simulink model "link"  (R2025b)
settings: Solver=FixedStepAuto  StartTime=0.0  StopTime=10.0  RelTol=1e-3
undefined symbols (not defined in the file): link_params, Ts_inner
settings Model: DataDictionary=project.sldd  Creator=Nick  LastModifiedBy=Nick

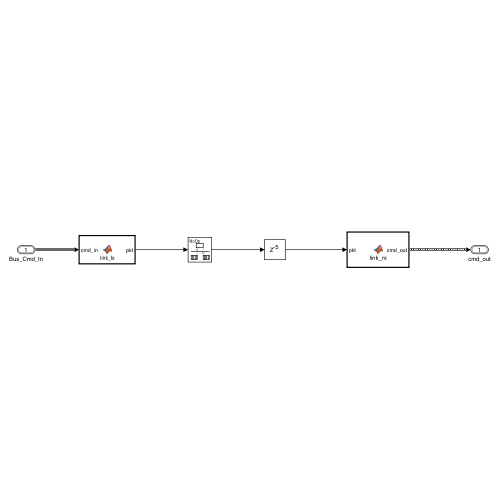
[thumbnail: Simulink's stored preview of the top-level diagram]
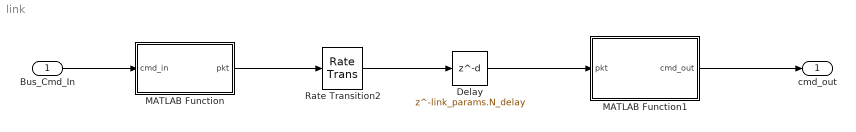
== system link ==
  Bus_Cmd_In : Inport  OutDataTypeStr=Bus: Bus_Cmd
  Delay : Delay  DelayLength=link_params.N_delay  InitialCondition=link_params.pkt_init_delay  SampleTime=Ts_inner
  MATLAB Function : MATLAB Function  TreatAsAtomicUnit=on
  MATLAB Function1 : MATLAB Function  TreatAsAtomicUnit=on
  Rate Transition2 : RateTransition  OutPortSampleTime=Ts_sim
  cmd_out : Outport  OutDataTypeStr=Bus: Bus_Cmd
  wires:
  Bus_Cmd_In/1 -> MATLAB Function/1(cmd_in)
  MATLAB Function/1(pkt) -> Rate Transition2/1
  Rate Transition2/1 -> Delay/1
  Delay/1 -> MATLAB Function1/1(pkt)
  MATLAB Function1/1(cmd_out) -> cmd_out/1

== matlab function link/MATLAB Function1 ==
  data: pkt input int16 size=[19 1]; link_params parameter; cmd_out output Bus: Bus_Cmd
function cmd_out = link_rx(pkt, link_params)
%#codegen
% RX-Seite Funkkanal (Drohne) @ Ts_inner.
%   int16-Paket (19x1) -> dequantisieren -> Bus_Cmd
%   Quaternionen werden re-normiert (Quant-Rauschen entfernen).
p    = reshape(double(pkt), 19, 1);
fs   = reshape(double(link_params.fs), 19, 1);
qmax = double(link_params.qmax);
lsb  = fs / qmax;
v    = reshape(p .* lsb, 19, 1);
F    = v(1);
qd   = reshape(v(2:5),   4, 1);
qr   = reshape(v(6:9),   4, 1);
Om   = reshape(v(10:12), 3, 1);
tr   = reshape(v(13:15), 3, 1);
qe   = reshape(v(16:19), 4, 1);
n_qd = sqrt(qd.'*qd); if n_qd < 1e-12, n_qd = 1; end
n_qr = sqrt(qr.'*qr); if n_qr < 1e-12, n_qr = 1; end
n_qe = sqrt(qe.'*qe); if n_qe < 1e-12, n_qe = 1; end
cmd_out.F_des     = F;
cmd_out.q_des     = qd / n_qd;
cmd_out.q_ref     = qr / n_qr;
cmd_out.Omega_ref = Om;
cmd_out.tau_ref   = tr;
cmd_out.q_ext     = qe / n_qe;
end

== matlab function link/MATLAB Function ==
  data: cmd_in input Bus: Bus_Cmd; pkt output int16 size=[19 1]; link_params parameter
function pkt = link_tx(cmd_in, link_params)
%#codegen
% TX-Seite Funkkanal (GCS->Drohne) @ Ts_gcs.
%   (1) Bus_Cmd -> 19x1 double in fester Reihenfolge packen
%   (2) int16-Quantisierung mit Saturierung
%   (3) Bernoulli-Paketverlust (xorshift32); bei Verlust letztes Paket halten (ZOH).
persistent last_pkt rs init_done
if isempty(init_done)
    last_pkt  = reshape(int16(link_params.pkt_init), 19, 1);
    rs        = uint32(link_params.seed);
    init_done = true;
end
F   = double(cmd_in.F_des);
qd  = reshape(double(cmd_in.q_des),     4, 1);
qr  = reshape(double(cmd_in.q_ref),     4, 1);
Om  = reshape(double(cmd_in.Omega_ref), 3, 1);
tr  = reshape(double(cmd_in.tau_ref),   3, 1);
qe  = reshape(double(cmd_in.q_ext),     4, 1);
v   = reshape([F; qd; qr; Om; tr; qe], 19, 1);
fs   = reshape(double(link_params.fs), 19, 1);
qmax = double(link_params.qmax);
qmin = double(link_params.qmin);
lsb  = fs / qmax;
qi      = min(max(round(v ./ lsb), qmin), qmax);
pkt_now = reshape(int16(qi), 19, 1);
[u, rs] = xorshift01(rs);
if u >= link_params.pdrop
    last_pkt = pkt_now;
end
pkt = reshape(last_pkt, 19, 1);
end
function [u, s] = xorshift01(s)
% xorshift32 -> u in [0,1). Seed != 0 erforderlich.
s = bitxor(s, bitshift(s,  13));
s = bitxor(s, bitshift(s, -17));
s = bitxor(s, bitshift(s,   5));
u = double(s) / 4294967296;
end
